simulink model "ReglerVergleich"  (R2021b)
settings: Solver=VariableStepAuto  StartTime=0.0  StopTime=53  RelTol=1e-3
values from neighbouring files (symbols this model uses):
  sampleTime = 0.01    [EchtwertVergleichSkript.m]    (also in ReglerVergleich_.m = max(M.Time)/length(M.Time))
settings Model: Creator=tim  LastModifiedBy=tim

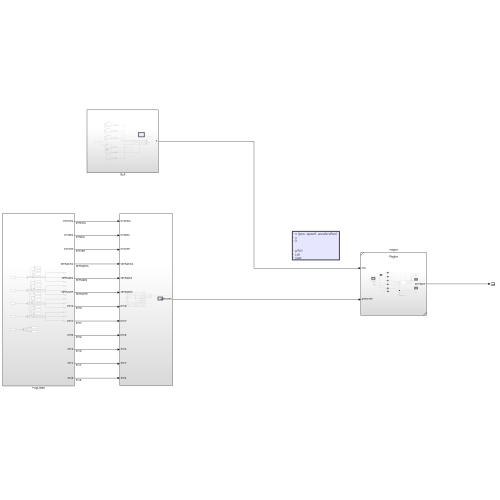
[thumbnail: Simulink's stored preview of the top-level diagram]
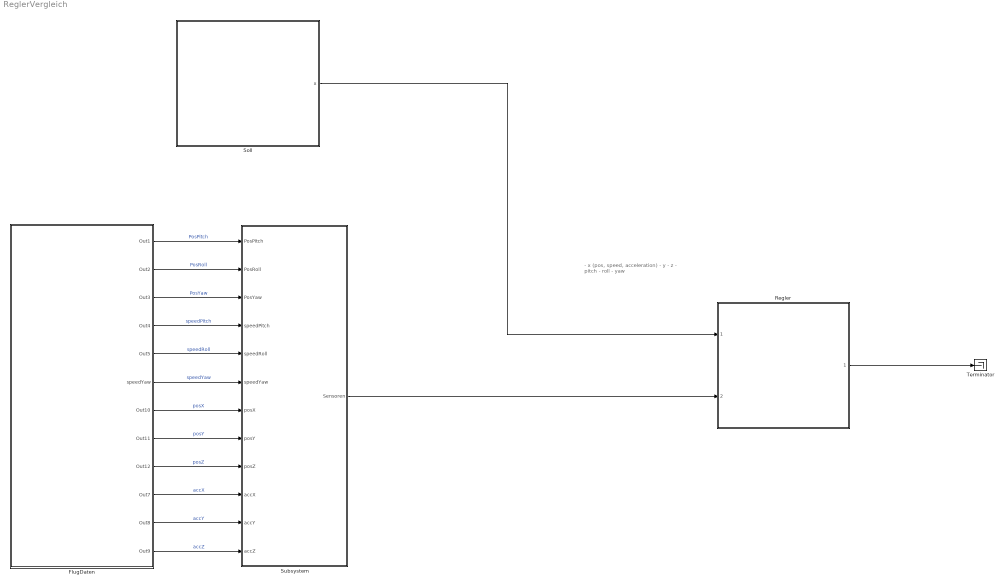
== system ReglerVergleich ==
  note: - x (pos, speed, acceleration)
      | - y
      | - z
      |
      |
      | - pitch
      | - roll
      | - yaw
  FlugDaten : Subsystem
  Regler : Subsystem  VariantControl=Choice  ReferencedSubsystem=Regler
  Soll : Subsystem
  Subsystem : Subsystem
  Terminator : Terminator
  wires:
  Soll/1(x) -> Regler/1
  FlugDaten/1(Out1) -> Subsystem/1(PosPitch)  "PosPitch"
  FlugDaten/2(Out2) -> Subsystem/2(PosRoll)  "PosRoll"
  FlugDaten/3(Out3) -> Subsystem/3(PosYaw)  "PosYaw"
  FlugDaten/4(Out4) -> Subsystem/4(speedPitch)  "speedPitch"
  FlugDaten/5(Out5) -> Subsystem/5(speedRoll)  "speedRoll"
  FlugDaten/6(speedYaw) -> Subsystem/6(speedYaw)  "speedYaw"
  FlugDaten/7(Out10) -> Subsystem/7(posX)  "posX"
  FlugDaten/8(Out11) -> Subsystem/8(posY)  "posY"
  FlugDaten/9(Out12) -> Subsystem/9(posZ)  "posZ"
  FlugDaten/10(Out7) -> Subsystem/10(accX)  "accX"
  FlugDaten/11(Out8) -> Subsystem/11(accY)  "accY"
  FlugDaten/12(Out9) -> Subsystem/12(accZ)  "accZ"
  Subsystem/1(Sensoren) -> Regler/2
  Regler/1 -> Terminator/1

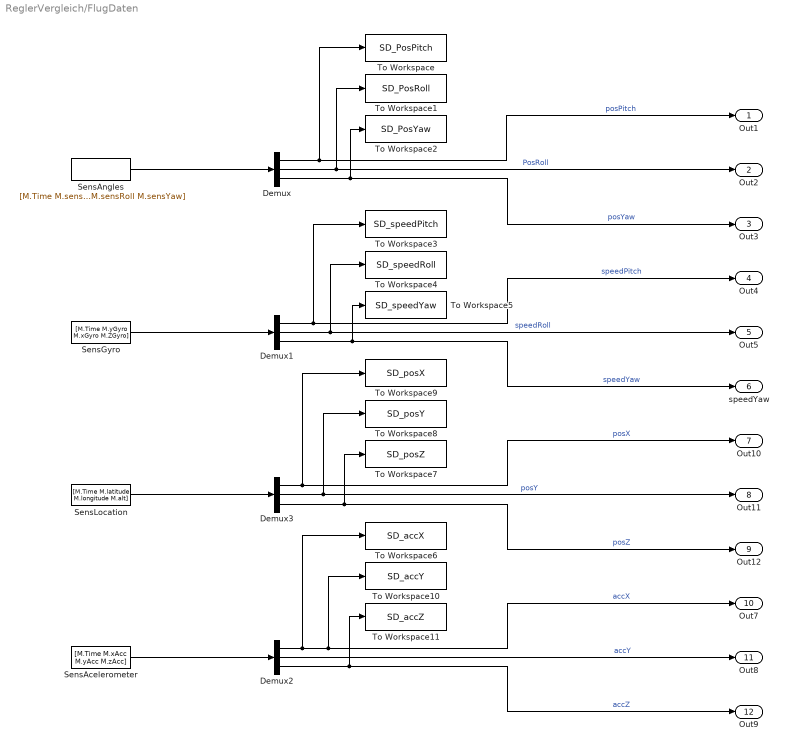
== system ReglerVergleich/FlugDaten ==
  Demux{,1..3} (4 alike) : Demux  Outputs=3
  SensAcelerometer : FromWorkspace  VariableName=[M.Time M.xAcc M.yAcc M.zAcc]  SampleTime=sampleTime  Interpolate=off  OutputAfterFinalValue=Holding final value
  SensAngles : FromWorkspace  VariableName=[M.Time M.sensPitch M.sensRoll M.sensYaw]  SampleTime=sampleTime  Interpolate=off  OutputAfterFinalValue=Holding final value
  SensGyro : FromWorkspace  VariableName=[M.Time M.yGyro M.xGyro M.ZGyro]  SampleTime=sampleTime  Interpolate=off  OutputAfterFinalValue=Holding final value
  SensLocation : FromWorkspace  VariableName=[M.Time M.latitude M.longitude M.alt]  SampleTime=sampleTime  Interpolate=off  OutputAfterFinalValue=Holding final value
  To Workspace : ToWorkspace  VariableName=SD_PosPitch  SaveFormat=Timeseries  SampleTime=-1
  To Workspace1 : ToWorkspace  VariableName=SD_PosRoll  SaveFormat=Timeseries  SampleTime=-1
  To Workspace10 : ToWorkspace  VariableName=SD_accY  SaveFormat=Timeseries  SampleTime=-1
  To Workspace11 : ToWorkspace  VariableName=SD_accZ  SaveFormat=Timeseries  SampleTime=-1
  To Workspace2 : ToWorkspace  VariableName=SD_PosYaw  SaveFormat=Timeseries  SampleTime=-1
  To Workspace3 : ToWorkspace  VariableName=SD_speedPitch  SaveFormat=Timeseries  SampleTime=-1
  To Workspace4 : ToWorkspace  VariableName=SD_speedRoll  SaveFormat=Timeseries  SampleTime=-1
  To Workspace5 : ToWorkspace  VariableName=SD_speedYaw  SaveFormat=Timeseries  SampleTime=-1
  To Workspace6 : ToWorkspace  VariableName=SD_accX  SaveFormat=Timeseries  SampleTime=-1
  To Workspace7 : ToWorkspace  VariableName=SD_posZ  SaveFormat=Timeseries  SampleTime=-1
  To Workspace8 : ToWorkspace  VariableName=SD_posY  SaveFormat=Timeseries  SampleTime=-1
  To Workspace9 : ToWorkspace  VariableName=SD_posX  SaveFormat=Timeseries  SampleTime=-1
  Out1 : Outport
  Out2 : Outport  Port=2
  Out3 : Outport  Port=3
  Out4 : Outport  Port=4
  Out5 : Outport  Port=5
  speedYaw : Outport  Port=6
  Out10 : Outport  Port=7
  Out11 : Outport  Port=8
  Out12 : Outport  Port=9
  Out7 : Outport  Port=10
  Out8 : Outport  Port=11
  Out9 : Outport  Port=12
  wires:
  Demux/1 -> To Workspace/1, Out1/1  "posPitch"
  Demux/2 -> To Workspace1/1, Out2/1  "PosRoll"
  Demux/3 -> To Workspace2/1, Out3/1  "posYaw"
  Demux1/2 -> To Workspace4/1, Out5/1  "speedRoll"
  Demux2/2 -> Out8/1  "accY"
  Demux2/1 -> To Workspace6/1, To Workspace10/1, Out7/1  "accX"
  Demux2/3 -> To Workspace11/1, Out9/1  "accZ"
  Demux1/3 -> To Workspace5/1, speedYaw/1  "speedYaw"
  Demux1/1 -> To Workspace3/1, Out4/1  "speedPitch"
  Demux3/1 -> To Workspace9/1, Out10/1  "posX"
  Demux3/2 -> To Workspace8/1, Out11/1  "posY"
  Demux3/3 -> To Workspace7/1, Out12/1  "posZ"
  SensAcelerometer/1 -> Demux2/1
  SensLocation/1 -> Demux3/1
  SensAngles/1 -> Demux/1
  SensGyro/1 -> Demux1/1

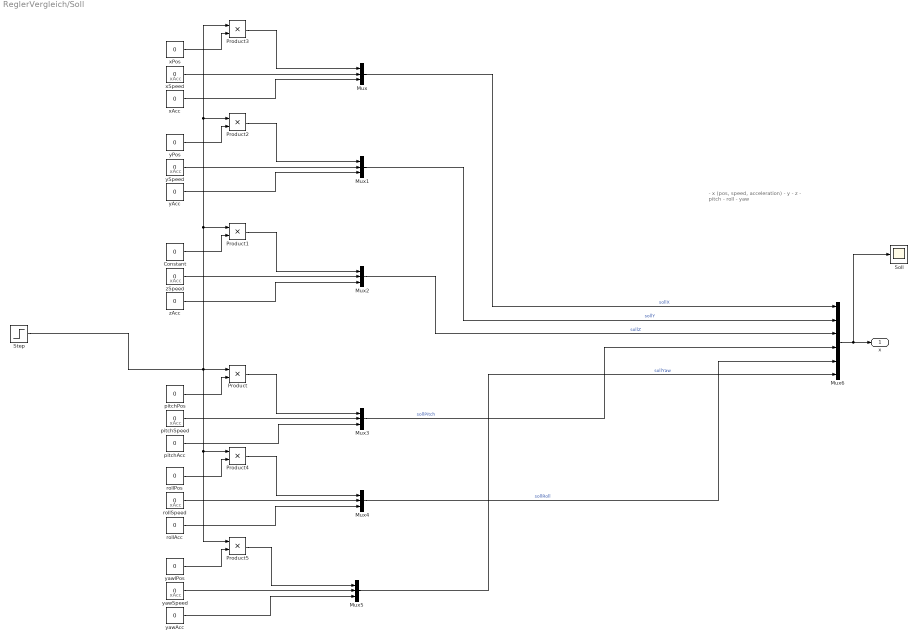
== system ReglerVergleich/Soll ==
  note: - x (pos, speed, acceleration)
      | - y
      | - z
      |
      |
      | - pitch
      | - roll
      | - yaw
  note: xAcc
  note: xAcc
  note: xAcc
  note: xAcc
  note: xAcc
  note: xAcc
  Constant : Constant  Value=0
  Mux{,1..5} (6 alike) : Mux  Inputs=3
  Mux6 : Mux  Inputs=6
  Product{,1..5} (6 alike) : Product
  Soll : Scope
  Step : Step  SampleTime=0
  pitchAcc : Constant  Value=0
  pitchPos : Constant  Value=0
  pitchSpeed : Constant  Value=0
  rollAcc : Constant  Value=0
  rollPos : Constant  Value=0
  rollSpeed : Constant  Value=0
  xAcc : Constant  Value=0
  xPos : Constant  Value=0
  xSpeed : Constant  Value=0
  yAcc : Constant  Value=0
  yPos : Constant  Value=0
  ySpeed : Constant  Value=0
  yawAcc : Constant  Value=0
  yawSpeed : Constant  Value=0
  yawlPos : Constant  Value=0
  zAcc : Constant  Value=0
  zSpeed : Constant  Value=0
  x : Outport
  wires:
  Mux/1 -> Mux6/1  "sollX"
  Mux1/1 -> Mux6/2  "sollY"
  Mux2/1 -> Mux6/3  "sollZ"
  Mux4/1 -> Mux6/5  "sollRoll"
  Mux5/1 -> Mux6/6  "sollYaw"
  Mux3/1 -> Mux6/4  "sollPitch"
  Mux6/1 -> Soll/1, x/1
  pitchAcc/1 -> Mux3/3
  pitchSpeed/1 -> Mux3/2
  Product/1 -> Mux3/1
  pitchPos/1 -> Product/2
  zAcc/1 -> Mux2/3
  zSpeed/1 -> Mux2/2
  Product1/1 -> Mux2/1
  Constant/1 -> Product1/2
  yAcc/1 -> Mux1/3
  ySpeed/1 -> Mux1/2
  Product2/1 -> Mux1/1
  yPos/1 -> Product2/2
  xAcc/1 -> Mux/3
  xSpeed/1 -> Mux/2
  Product3/1 -> Mux/1
  xPos/1 -> Product3/2
  rollAcc/1 -> Mux4/3
  rollSpeed/1 -> Mux4/2
  Product4/1 -> Mux4/1
  rollPos/1 -> Product4/2
  yawlPos/1 -> Product5/2
  yawSpeed/1 -> Mux5/2
  yawAcc/1 -> Mux5/3
  Product5/1 -> Mux5/1
  Step/1 -> Product3/1, Product2/1, Product1/1, Product5/1, Product4/1, Product/1

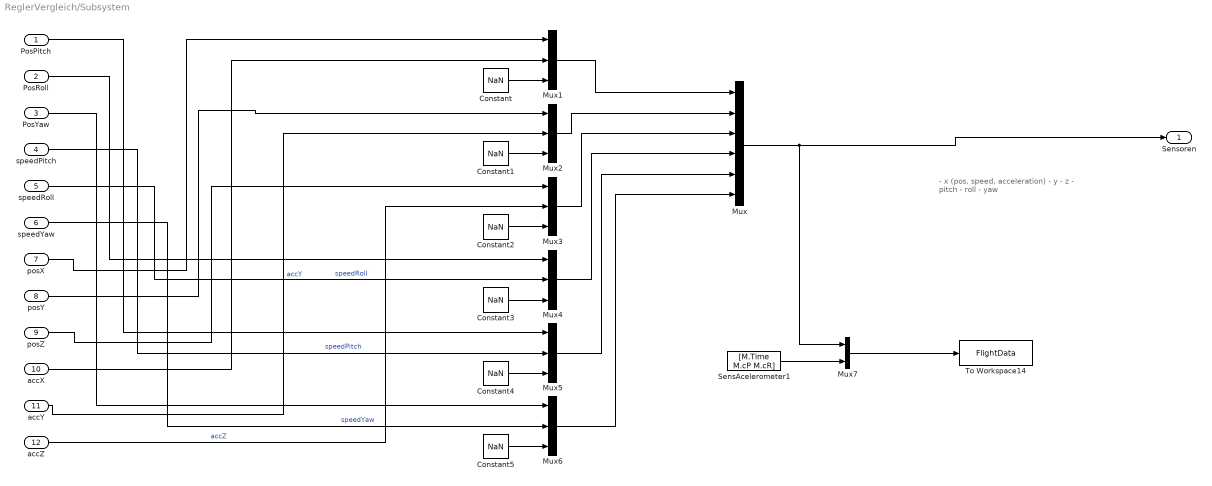
== system ReglerVergleich/Subsystem ==
  note: - x (pos, speed, acceleration)
      | - y
      | - z
      |
      |
      | - pitch
      | - roll
      | - yaw
  PosPitch : Inport
  PosRoll : Inport  Port=2
  PosYaw : Inport  Port=3
  speedPitch : Inport  Port=4
  speedRoll : Inport  Port=5
  speedYaw : Inport  Port=6
  posX : Inport  Port=7
  posY : Inport  Port=8
  posZ : Inport  Port=9
  accX : Inport  Port=10
  accY : Inport  Port=11
  accZ : Inport  Port=12
  Constant{,1..5} (6 alike) : Constant  Value=NaN
  Mux : Mux  Inputs=6
  Mux{1..6} (6 alike) : Mux  Inputs=3
  Mux7 : Mux  Inputs=2
  SensAcelerometer1 : FromWorkspace  VariableName=[M.Time M.cP M.cR]  SampleTime=sampleTime  Interpolate=off  OutputAfterFinalValue=Holding final value
  To Workspace14 : ToWorkspace  VariableName=FlightData  SaveFormat=Timeseries  SampleTime=-1
  Sensoren : Outport
  wires:
  Mux1/1 -> Mux/1
  Mux2/1 -> Mux/2
  Mux3/1 -> Mux/3
  PosYaw/1 -> Mux6/1
  PosPitch/1 -> Mux5/1
  PosRoll/1 -> Mux4/1
  speedPitch/1 -> Mux5/2  "speedPitch"
  speedRoll/1 -> Mux4/2  "speedRoll"
  speedYaw/1 -> Mux6/2  "speedYaw"
  posX/1 -> Mux1/1
  posY/1 -> Mux2/1
  posZ/1 -> Mux3/1
  accX/1 -> Mux1/2
  accY/1 -> Mux2/2  "accY"
  accZ/1 -> Mux3/2  "accZ"
  Mux/1 -> Sensoren/1, Mux7/1
  Mux4/1 -> Mux/4
  Mux5/1 -> Mux/5
  Mux6/1 -> Mux/6
  Constant/1 -> Mux1/3
  Constant1/1 -> Mux2/3
  Constant2/1 -> Mux3/3
  Constant3/1 -> Mux4/3
  Constant4/1 -> Mux5/3
  Constant5/1 -> Mux6/3
  Mux7/1 -> To Workspace14/1
  SensAcelerometer1/1 -> Mux7/2
